simulink model "PID_Validation"  (R2024b)
settings: Solver=ode45  StartTime=0.0  StopTime=10.0  RelTol=1e-3
InitFcn:
  | Init
values from neighbouring files (symbols this model uses):
  Kd = Kp * Td    [Init.m]    (also in code.m; main.m)
  Ki = Kp / Ti    [Init.m]    (also in code.m; main.m)
  Kp = deltak * cos(deltaphi)    [Init.m]    (also in code.m = deltak*cos(deltaphi); main.m = deltak*cos(deltaphi))
  tl = 1/(3*wgc)    [Init.m]    (also in code.m = 1/cut_off; main.m = 1/cut_off)
undefined symbols (not defined in the file or in its folder): drv, gbox, mld, mot, sens
libraries: simulink_extras x1
settings Model: Creator=Banaan  LastModifiedBy=lucag

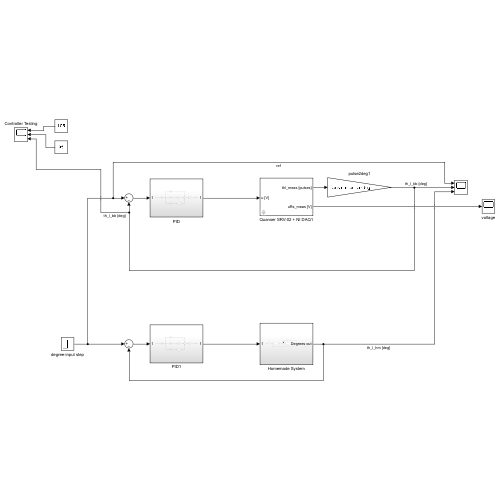
[thumbnail: Simulink's stored preview of the top-level diagram]
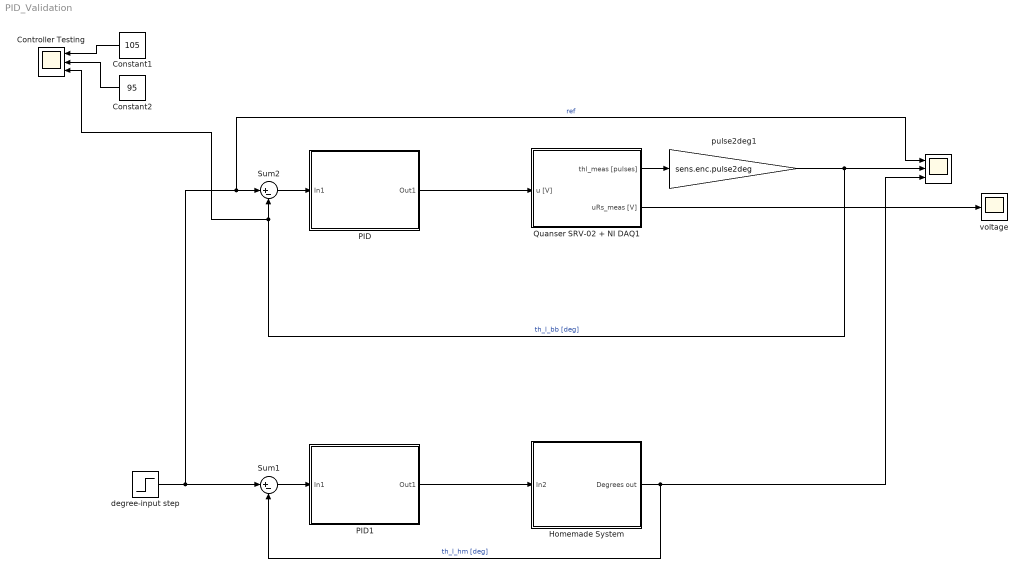
== system PID_Validation ==
  " " : Scope  NumInputPorts=3
  Constant1 : Constant  Value=105
  Constant2 : Constant  Value=95
  Controller Testing : Scope  NumInputPorts=3
  Homemade System : Subsystem
  PID : Subsystem
  PID1 : Subsystem
  Quanser SRV-02 + NI DAQ1 : Subsystem  mask(Quanser SRV-02 (with inertial load) + NI DAQ){Ts=0.001, fricType=Coulomb + viscous}
      mask prompts: Ts "NI DAQ Sample Time:"; fricType "Friction model"
      mask help: Quanser SRV-02 (with inertial load) + NI DAQ model.
      mask init:
      | %%  Sensors data
      | 
      | %   shunt resistor
      | sens.curr.Rs = 0.5;                         %   resistance [Ohm]   
      | sens.curr.uRs_std = 0.01;                   %   voltage noise standard dev [V]                           
      | sens.curr.uRs_var = sens.curr.uRs_std^2;	%   voltage noise variance [V^2]
      | 
      | %   Hewlett-Packard HEDS-5540#A06 optical encoder
      | sens.enc.ppr = 500*4;                       %   pulses per rotation
      | sens.enc.pulse2deg = 360/sens.enc.ppr;      %   [pulses] -> [deg]
      | sens.enc.pulse2rad = 2*pi/sens.enc.ppr;     %   [pulses] -> [rad]
      | sens.enc.deg2pulse = sens.enc.ppr/360;      %   [deg] -> [pulses]
      | sens.enc.rad2pulse = sens.enc.ppr/2/pi;     %   [rad] -> [pulses]
      | 
      | 
      | %%  Data acquisition board (daq) data
      | 
      | %   NI PCI-6221 DAC data
      | daq.dac.bits = 16;                                  %   resolution (bits)
      | daq.dac.fs   = 10;                                  %   full scale 
      | daq.dac.q    = 2*daq.dac.fs/(2^daq.dac.bits-1);     %	quantization
      | 
      | %   NI PCI-6221 ADC data
      | daq.adc.bits = 16;                                  %   resolution (bits)
      | daq.adc.fs   = 10;                                  %   full scale (as set in SLDRT Analog Input block)
      | daq.adc.q    = 2*daq.adc.fs/(2^daq.adc.bits-1);     %   quantization
      mask Help:
      | Riccardo Antonello (antonello@dei.unipd.it)
      | 
      | April 24, 2020
      | 
      | Dept. of Information Engineering, University of Padova
      mask TypeOptions fricType: Coulomb + viscous | Karnopp
  Sum1 : Sum  Inputs=|+-
  Sum2 : Sum  Inputs=|+-
  degree-input step : Step  After=20  SampleTime=0
  pulse2deg1 : Gain  Gain=sens.enc.pulse2deg
  voltage : Scope
  wires:
  degree-input step/1 -> " "/1, Sum2/1, Sum1/1  "ref"
  Constant1/1 -> Controller Testing/1
  Sum2/1 -> PID/1(In1)
  Quanser SRV-02 + NI DAQ1/1(thl_meas [pulses]) -> pulse2deg1/1
  PID/1(Out1) -> Quanser SRV-02 + NI DAQ1/1(u [V])
  Constant2/1 -> Controller Testing/2
  Quanser SRV-02 + NI DAQ1/2(uRs_meas [V]) -> voltage/1
  pulse2deg1/1 -> Controller Testing/3, Sum2/2, " "/2  "th_l_bb [deg]"
  Sum1/1 -> PID1/1(In1)
  PID1/1(Out1) -> Homemade System/1(In2)
  Homemade System/1(Degrees out) -> " "/3, Sum1/2  "th_l_hm [deg]"

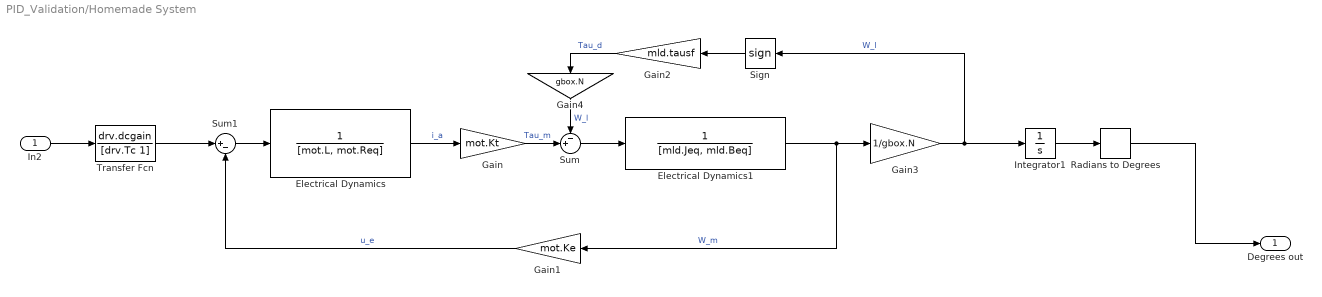
== system PID_Validation/Homemade System ==
  In2 : Inport
  Electrical Dynamics : TransferFcn  Denominator=[mot.L, mot.Req]
  Electrical Dynamics1 : TransferFcn  Denominator=[mld.Jeq, mld.Beq]
  Gain : Gain  Gain=mot.Kt
  Gain1 : Gain  Gain=mot.Ke
  Gain2 : Gain  Gain=mld.tausf
  Gain3 : Gain  Gain=1/gbox.N
  Gain4 : Gain  Gain=gbox.N
  Integrator1 : Integrator
  Radians to Degrees : simulink_extras/Transformations/Radians to Degrees
  Sign : Signum  ZeroCross=off
  Sum : Sum  Inputs=-+|
  Sum1 : Sum  Inputs=|+-
  Transfer Fcn : TransferFcn  Numerator=drv.dcgain  Denominator=[drv.Tc 1]
  Degrees out : Outport
  wires:
  Gain/1 -> Sum/2  "Tau_m"
  Electrical Dynamics1/1 -> Gain1/1, Gain3/1  "W_m"
  Integrator1/1 -> Radians to Degrees/1
  Gain3/1 -> Integrator1/1, Sign/1  "W_l"
  Sign/1 -> Gain2/1
  Gain1/1 -> Sum1/2  "u_e"
  Electrical Dynamics/1 -> Gain/1  "i_a"
  Gain4/1 -> Sum/1  "W_l"
  Sum/1 -> Electrical Dynamics1/1
  Gain2/1 -> Gain4/1  "Tau_d"
  Sum1/1 -> Electrical Dynamics/1
  Transfer Fcn/1 -> Sum1/1
  Radians to Degrees/1 -> Degrees out/1
  In2/1 -> Transfer Fcn/1

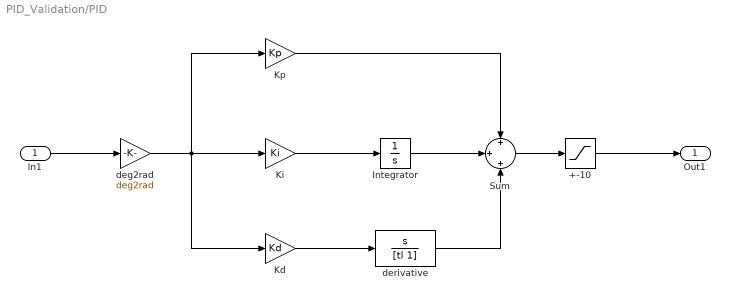
== system PID_Validation/PID ==
  In1 : Inport
  +-10 : Saturate  UpperLimit=10  LowerLimit=-10
  Integrator : Integrator
  Kd : Gain  Gain=Kd
  Ki : Gain  Gain=Ki
  Kp : Gain  Gain=Kp
  Sum : Sum  Inputs=+|+|+
  deg2rad : Gain  Gain=deg2rad
  derivative : TransferFcn  Numerator=[1 0]  Denominator=[tl 1]
  Out1 : Outport
  wires:
  In1/1 -> deg2rad/1
  deg2rad/1 -> Kd/1, Kp/1, Ki/1
  Ki/1 -> Integrator/1
  Kp/1 -> Sum/1
  Integrator/1 -> Sum/2
  Kd/1 -> derivative/1
  derivative/1 -> Sum/3
  Sum/1 -> +-10/1
  +-10/1 -> Out1/1

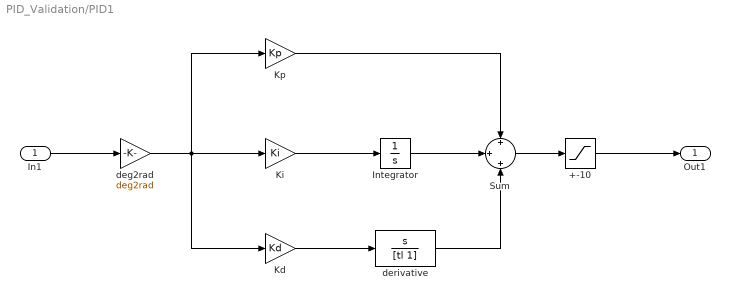
== system PID_Validation/PID1 ==
  In1 : Inport
  +-10 : Saturate  UpperLimit=10  LowerLimit=-10
  Integrator : Integrator
  Kd : Gain  Gain=Kd
  Ki : Gain  Gain=Ki
  Kp : Gain  Gain=Kp
  Sum : Sum  Inputs=+|+|+
  deg2rad : Gain  Gain=deg2rad
  derivative : TransferFcn  Numerator=[1 0]  Denominator=[tl 1]
  Out1 : Outport
  wires:
  +-10/1 -> Out1/1
  Sum/1 -> +-10/1
  derivative/1 -> Sum/3
  Kd/1 -> derivative/1
  Integrator/1 -> Sum/2
  Kp/1 -> Sum/1
  Ki/1 -> Integrator/1
  deg2rad/1 -> Ki/1, Kp/1, Kd/1
  In1/1 -> deg2rad/1

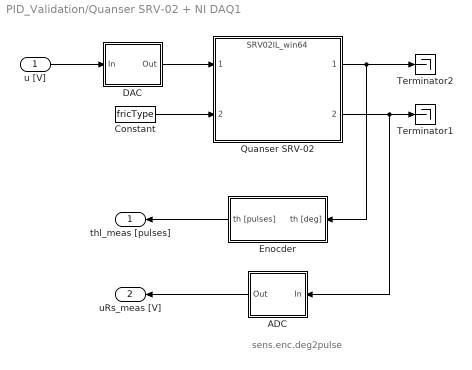
== system PID_Validation/Quanser SRV-02 + NI DAQ1 ==
  note: sens.enc.deg2pulse
  u [V] : Inport
  ADC : Subsystem
  Constant : Constant  Value=fricType
  DAC : Subsystem
  Enocder : Subsystem
  Quanser SRV-02 : ModelReference  ModelNameDialog=SRV02IL_win64.slxp  ModelReferenceVersion=1.44  CopyOfModelProtected=on
  Terminator1 : Terminator
  Terminator2 : Terminator
  thl_meas [pulses] : Outport
  uRs_meas [V] : Outport  Port=2
  wires:
  Enocder/1(th [pulses]) -> thl_meas [pulses]/1
  ADC/1(Out) -> uRs_meas [V]/1
  DAC/1(Out) -> Quanser SRV-02/1
  Quanser SRV-02/2 -> ADC/1(In), Terminator1/1
  u [V]/1 -> DAC/1(In)
  Quanser SRV-02/1 -> Enocder/1(th [deg]), Terminator2/1
  Constant/1 -> Quanser SRV-02/2

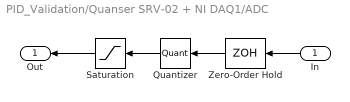
== system PID_Validation/Quanser SRV-02 + NI DAQ1/ADC ==
  In : Inport
  Quantizer : Quantizer  QuantizationInterval=daq.adc.q
  Saturation : Saturate  UpperLimit=daq.adc.fs  LowerLimit=-daq.adc.fs
  Zero-Order Hold : ZeroOrderHold  SampleTime=Ts
  Out : Outport
  wires:
  Saturation/1 -> Out/1
  In/1 -> Zero-Order Hold/1
  Quantizer/1 -> Saturation/1
  Zero-Order Hold/1 -> Quantizer/1

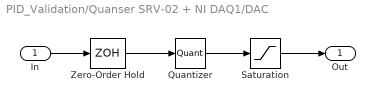
== system PID_Validation/Quanser SRV-02 + NI DAQ1/DAC ==
  In : Inport
  Quantizer : Quantizer  QuantizationInterval=daq.dac.q
  Saturation : Saturate  UpperLimit=daq.dac.fs  LowerLimit=-daq.dac.fs
  Zero-Order Hold : ZeroOrderHold  SampleTime=Ts
  Out : Outport
  wires:
  Quantizer/1 -> Saturation/1
  In/1 -> Zero-Order Hold/1
  Zero-Order Hold/1 -> Quantizer/1
  Saturation/1 -> Out/1

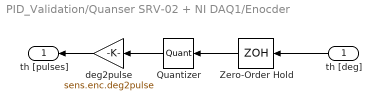
== system PID_Validation/Quanser SRV-02 + NI DAQ1/Enocder ==
  th [deg] : Inport
  Quantizer : Quantizer  QuantizationInterval=sens.enc.pulse2deg
  Zero-Order Hold : ZeroOrderHold  SampleTime=Ts
  deg2pulse : Gain  Gain=sens.enc.deg2pulse
  th [pulses] : Outport
  wires:
  Quantizer/1 -> deg2pulse/1
  th [deg]/1 -> Zero-Order Hold/1
  Zero-Order Hold/1 -> Quantizer/1
  deg2pulse/1 -> th [pulses]/1
